simulink model "newSimulink_design"  (R2018a)
settings: Solver=ode45  StartTime=0.0  StopTime=100.0  RelTol=1e-3
settings Model: Creator=muhsi  LastModifiedBy=muhsi

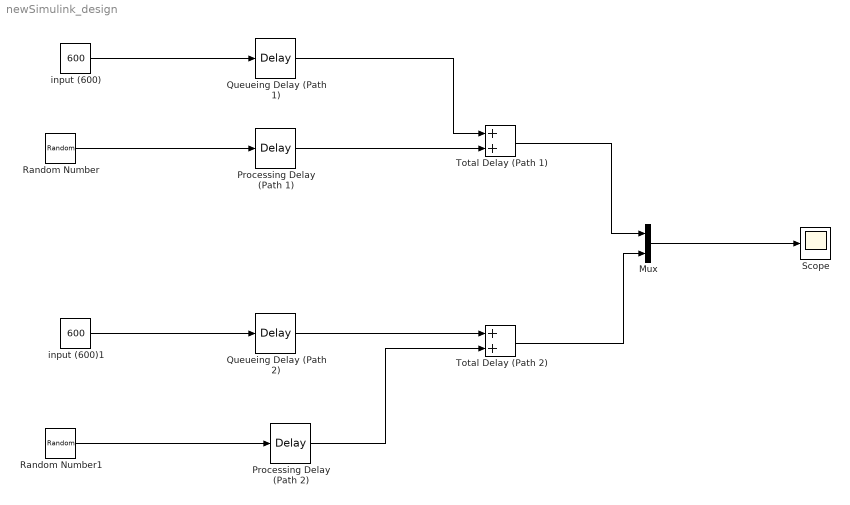
== system newSimulink_design ==
  Mux : Mux  Inputs=2
  Processing Delay (Path 1) : TransportDelay  DelayTime=154
  "Processing Delay (Path 2) " : TransportDelay  DelayTime=84
  Queueing Delay (Path 1) : TransportDelay  DelayTime=289
  Queueing Delay (Path 2) : TransportDelay  DelayTime=47
  Random Number : RandomNumber  Mean=289  Variance=30.9  SampleTime=0.1
  Random Number1 : RandomNumber  Mean=84  Variance=20  SampleTime=0.1
  Scope : Scope
  Total Delay (Path 1) : Sum
  Total Delay (Path 2) : Sum
  input (600) : Constant  Value=600
  input (600)1 : Constant  Value=600
  wires:
  Queueing Delay (Path 1)/1 -> Total Delay (Path 1)/1
  Processing Delay (Path 1)/1 -> Total Delay (Path 1)/2
  Queueing Delay (Path 2)/1 -> Total Delay (Path 2)/1
  "Processing Delay (Path 2) "/1 -> Total Delay (Path 2)/2
  Total Delay (Path 1)/1 -> Mux/1
  Total Delay (Path 2)/1 -> Mux/2
  Mux/1 -> Scope/1
  input (600)/1 -> Queueing Delay (Path 1)/1
  input (600)1/1 -> Queueing Delay (Path 2)/1
  Random Number/1 -> Processing Delay (Path 1)/1
  Random Number1/1 -> "Processing Delay (Path 2) "/1
